simulink model "NotchDLeadLag"  (R2025b)
settings: Solver=VariableStepAuto  StartTime=0.0  StopTime=10.0  RelTol=1e-3
values from neighbouring files (symbols this model uses):
  a = 7.8824697    [ControllerDesign.m]
  b = 79.28987    [ControllerDesign.m]
  b1 = 0.0257    [ControllerDesign.m]
  b2 = 0.0026    [ControllerDesign.m]
  C = 0.000    (= 0)    [ControllerDesign.m]
  c = 10    [ControllerDesign.m]
  d = 0.1    [ControllerDesign.m]
  d1 = 0.5431    [ControllerDesign.m]
  d2 = 0.0543    [ControllerDesign.m]
  k = 0.025    [ControllerDesign.m]
  Kp = K_Val{i}    [ControllerDesign.m]
  m1 = 0.00031231    [ControllerDesign.m]
  m2 = 0.00016865    [ControllerDesign.m]
  wn = 15.245    [ControllerDesign.m]
  zeta = sqrt(2)    [ControllerDesign.m]
settings Model: Creator=mthan  LastModifiedBy=mthan

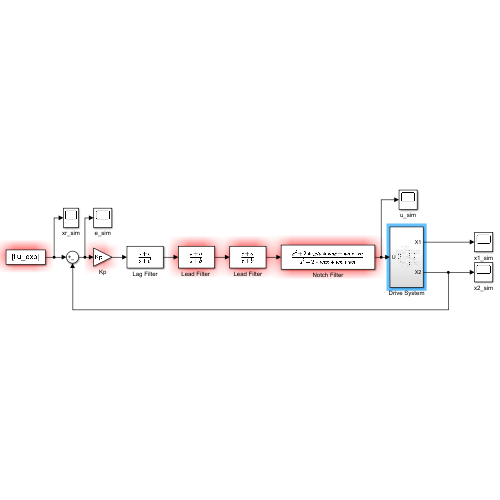
[thumbnail: Simulink's stored preview of the top-level diagram]
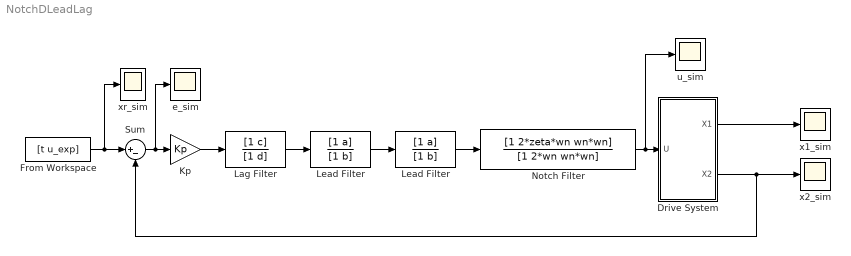
== system NotchDLeadLag ==
  Drive System : Subsystem
  From Workspace : FromWorkspace  VariableName=[t u_exp]
  Kp : Gain  Gain=Kp
  Lag Filter : TransferFcn  Numerator=[1 c]  Denominator=[1 d]
  Lead Filter : TransferFcn  Numerator=[1 a]  Denominator=[1 b]
  "Lead Filter " : TransferFcn  Numerator=[1 a]  Denominator=[1 b]
  Notch Filter : TransferFcn  Numerator=[1 2*zeta*wn wn*wn]  Denominator=[1 2*wn wn*wn]
  Sum : Sum  Inputs=|+-
  e_sim : Scope
      settings: DataLoggingVariableName=e_sim  DataLoggingSaveFormat=Array
  u_sim : Scope
      settings: DataLoggingVariableName=u_sim  DataLoggingSaveFormat=Array
  x1_sim : Scope
      settings: DataLoggingVariableName=x1_sim  DataLoggingSaveFormat=Array
  x2_sim : Scope
      settings: DataLoggingVariableName=x2_sim  DataLoggingSaveFormat=Array
  xr_sim : Scope
      settings: DataLoggingVariableName=xr_sim  DataLoggingSaveFormat=Array
  wires:
  "Lead Filter "/1 -> Lead Filter/1
  Lead Filter/1 -> Notch Filter/1
  Notch Filter/1 -> u_sim/1, Drive System/1(U)
  Sum/1 -> e_sim/1, Kp/1
  From Workspace/1 -> xr_sim/1, Sum/1
  Drive System/1(X1) -> x1_sim/1
  Drive System/2(X2) -> Sum/2, x2_sim/1
  Kp/1 -> Lag Filter/1
  Lag Filter/1 -> "Lead Filter "/1

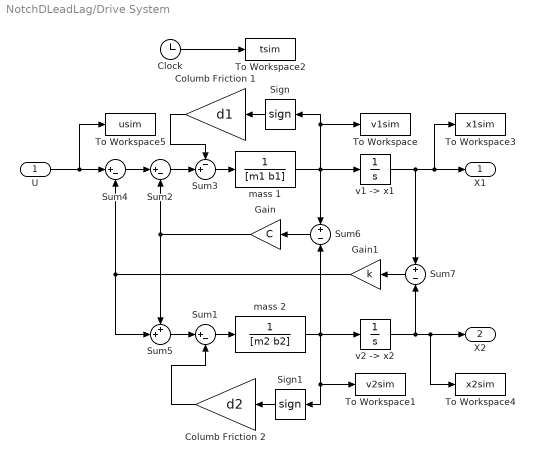
== system NotchDLeadLag/Drive System ==
  U : Inport
  Clock : Clock
  Columb Friction 1 : Gain  Gain=d1
  Columb Friction 2 : Gain  Gain=d2
  Gain : Gain  Gain=C  SaturateOnIntegerOverflow=on  OutDataTypeStr=Inherit: Same as input  ParamDataTypeStr=Inherit: Same as input
  Gain1 : Gain  Gain=k  SaturateOnIntegerOverflow=on  OutDataTypeStr=Inherit: Same as input  ParamDataTypeStr=Inherit: Same as input
  Sign : Signum
  Sign1 : Signum
  Sum1 : Sum  Inputs=|+-  SaturateOnIntegerOverflow=on
  Sum2 : Sum  Inputs=|+-  SaturateOnIntegerOverflow=on
  Sum3 : Sum  Inputs=-+|  SaturateOnIntegerOverflow=on
  Sum4 : Sum  Inputs=|+-  SaturateOnIntegerOverflow=on
  Sum5 : Sum  Inputs=++|  SaturateOnIntegerOverflow=on
  Sum6 : Sum  Inputs=+|-  SaturateOnIntegerOverflow=on
  Sum7 : Sum  Inputs=+|-  SaturateOnIntegerOverflow=on
  To Workspace : ToWorkspace  VariableName=v1sim  SampleTime=-1
      settings: Save2DSignal=2-D array (concatenate along first dimension)
  To Workspace1 : ToWorkspace  VariableName=v2sim  SampleTime=-1
      settings: Save2DSignal=2-D array (concatenate along first dimension)
  To Workspace2 : ToWorkspace  VariableName=tsim  SampleTime=-1
  To Workspace3 : ToWorkspace  VariableName=x1sim  SampleTime=-1
      settings: Save2DSignal=2-D array (concatenate along first dimension)
  To Workspace4 : ToWorkspace  VariableName=x2sim  SampleTime=-1
      settings: Save2DSignal=2-D array (concatenate along first dimension)
  To Workspace5 : ToWorkspace  VariableName=usim  SampleTime=-1
  mass 1 : TransferFcn  Denominator=[m1 b1]
  mass 2 : TransferFcn  Denominator=[m2 b2]
  "v1 -> x1" : Integrator
  "v2 -> x2" : Integrator
  X1 : Outport
  X2 : Outport  Port=2
  wires:
  Sum2/1 -> Sum3/2
  mass 2/1 -> Sign1/1, To Workspace1/1, Sum6/2, "v2 -> x2"/1
  Columb Friction 1/1 -> Sum3/1
  mass 1/1 -> Sign/1, To Workspace/1, "v1 -> x1"/1, Sum6/1
  Sum6/1 -> Gain/1
  Sum5/1 -> Sum1/1
  "v2 -> x2"/1 -> Sum7/2, X2/1, To Workspace4/1
  Sum7/1 -> Gain1/1
  Sign/1 -> Columb Friction 1/1
  Clock/1 -> To Workspace2/1
  U/1 -> To Workspace5/1, Sum4/1
  "v1 -> x1"/1 -> Sum7/1, X1/1, To Workspace3/1
  Gain1/1 -> Sum4/2, Sum5/2
  Columb Friction 2/1 -> Sum1/2
  Sum3/1 -> mass 1/1
  Sum1/1 -> mass 2/1
  Sign1/1 -> Columb Friction 2/1
  Gain/1 -> Sum2/2, Sum5/1
  Sum4/1 -> Sum2/1
